simulink model "Lookup_table_processing"  (R2025b)
settings: Solver=VariableStepAuto  StartTime=0.0  StopTime=10.0  RelTol=1e-3
InitFcn:
  | Relation
values from neighbouring files (symbols this model uses):
  deflection = deflection_min:0.01:deflection_max    [Relation.m]
  extension = sqrt(a^2 + r^2 - 2.*a.*r.*cos(deg2rad(alpha-deflection))) - d    [Relation.m]
  F_act = M_pivot ./ lever_arm_actuator    [Relation.m]
  velocity = 300    [Relation.m]
settings Model: Creator=Arseni  LastModifiedBy=User

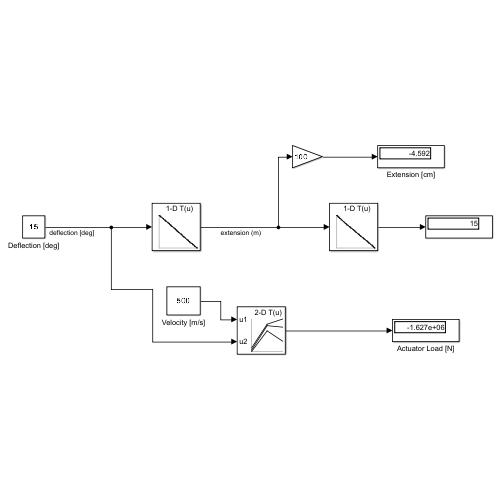
[thumbnail: Simulink's stored preview of the top-level diagram]
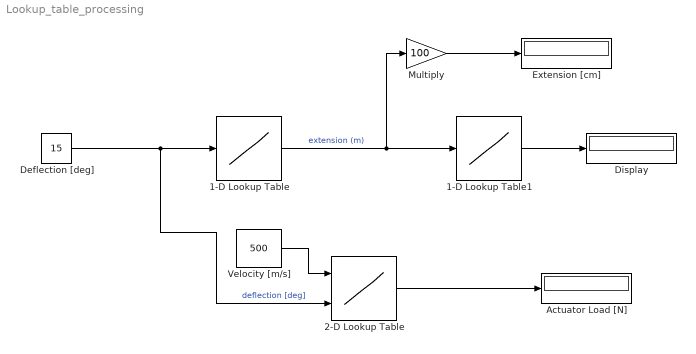
== system Lookup_table_processing ==
  1-D Lookup Table : Lookup_n-D  NumberOfTableDimensions=1  BreakpointsForDimension1=deflection  Table=extension  InternalRulePriority=Speed  RndMeth=Simplest
  1-D Lookup Table1 : Lookup_n-D  NumberOfTableDimensions=1  BreakpointsForDimension1=flip(extension)  Table=flip(deflection)  InternalRulePriority=Speed  RndMeth=Simplest
  2-D Lookup Table : Lookup_n-D  BreakpointsForDimension1=velocity  BreakpointsForDimension2=deflection  Table=F_act  InternalRulePriority=Speed  RndMeth=Simplest
      settings: InputPortMap=u0,u1
  Actuator Load [N] : Display
  Deflection [deg] : Constant  Value=15
  Display : Display
  Extension [cm] : Display
  Multiply : Gain  Gain=100
  Velocity [m/s] : Constant  Value=500
  wires:
  Deflection [deg]/1 -> 2-D Lookup Table/2, 1-D Lookup Table/1  "deflection [deg]"
  1-D Lookup Table/1 -> Multiply/1, 1-D Lookup Table1/1  "extension (m)"
  1-D Lookup Table1/1 -> Display/1
  Multiply/1 -> Extension [cm]/1
  2-D Lookup Table/1 -> Actuator Load [N]/1
  Velocity [m/s]/1 -> 2-D Lookup Table/1
